simulink model "Linear_Single_Model"  (R2022b)
settings: Solver=FixedStepAuto  StartTime=0.0  StopTime=10.0  FixedStep=0.01  RelTol=1e-3
values from neighbouring files (symbols this model uses):
  V = 30    [linearsinglemodel.m]
settings Model: Creator=FATMANURATA  LastModifiedBy=FATMANURATA

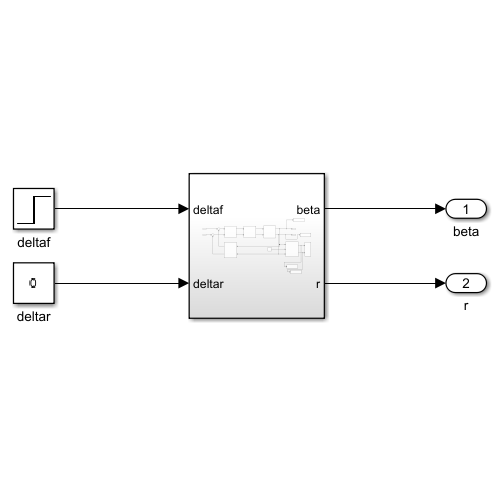
[thumbnail: Simulink's stored preview of the top-level diagram]
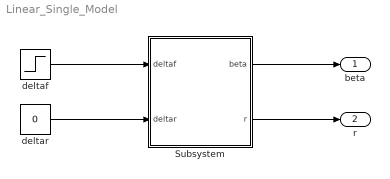
== system Linear_Single_Model ==
  Subsystem : Subsystem
  deltaf : Step  Time=0  SampleTime=0
  deltar : Constant  Value=0
  beta : Outport
  r : Outport  Port=2
  wires:
  deltaf/1 -> Subsystem/1(deltaf)
  deltar/1 -> Subsystem/2(deltar)
  Subsystem/1(beta) -> beta/1
  Subsystem/2(r) -> r/1

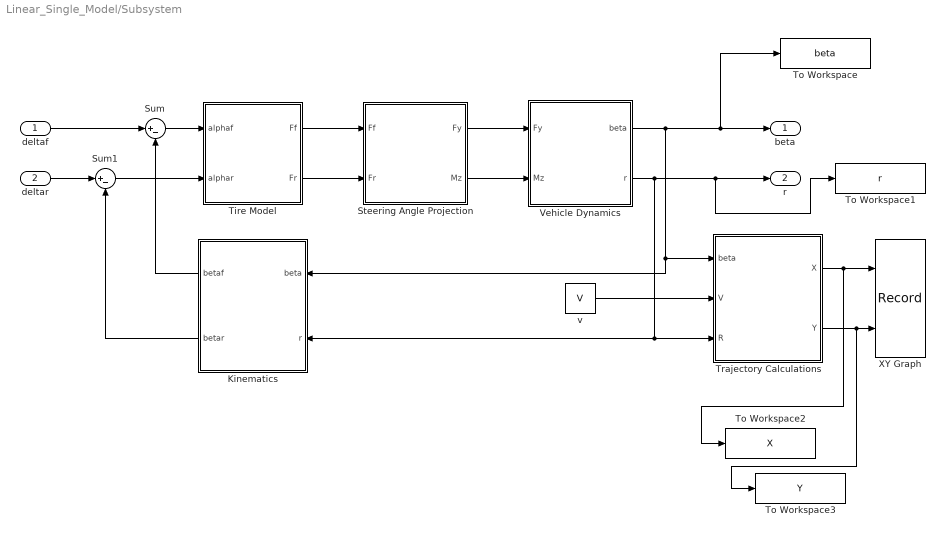
== system Linear_Single_Model/Subsystem ==
  deltaf : Inport
  deltar : Inport  Port=2
  Kinematics : Subsystem
  Steering Angle Projection : Subsystem
  Sum : Sum  Inputs=|+-
  Sum1 : Sum  Inputs=|+-
  Tire Model : Subsystem
  To Workspace : ToWorkspace  VariableName=beta  SampleTime=-1
  To Workspace1 : ToWorkspace  VariableName=r  SampleTime=-1
  To Workspace2 : ToWorkspace  VariableName=X  SampleTime=-1
  To Workspace3 : ToWorkspace  VariableName=Y  SampleTime=-1
  Trajectory Calculations : Subsystem
  Vehicle Dynamics : Subsystem
  XY Graph : Record  FileSettingsInternal="{\"entries\":[{\"content\":{\"excelSettings\":{\"content\":{},\"type\":\"Streamout.ExcelSettings\"}},\"type\":\"Streamout.FileSettingStorage\",\"uuid\":\"eae091c3-533e-4973-b4c9-77a1417e7f04\"}],\"packageUris\":[\"http://schema.mathworks.com/mf0/streamout_blocks/R2020a\"],\"version\":\"1.0\"}"  Layout=[1 1]  SignalsInternal="{\"entries\":[{\"content\":{\"signals\":[{\"content\":{\"blockPath\":[\"Linear_Single_Model/Subsystem/XY Graph\"],\"channel\":[],\"dimensions\":[1],\"domain\":\"Linear_Single_Model/Subsystem/XY Graph\",\"lineColor\":\"#b746ff\",\"plots\":[],\"port\":1,\"sid\":[\"\"],\"signalID\":1937,\"signalName\":\"Trajectory Calculations:1\"},\"type\":\"RecordBlkView.Signal\",\"uuid\":\"180f1f63-cad5-442e-bf7e-af3f779780d9\"},{\"content\":{\"blockPath\":[\"Linear_Single_Model/Subsystem/XY Graph\"],\"channel\":[],\"dimensions\":[1],\"domain\":\"Linear_Single_Model/Subsystem/XY Graph\",\"lineColor\":\"#64d413\",\"plots\":[],\"port\":2,\"sid\":[\"\"],\"signalID\":1941,\"signalName\":\"Trajectory Calculations:2\"},\"type\":\"RecordBlkView.Signal\",\"uuid\":\"a40823eb-ffdd-4da1-8b1e-2047577bc852\"}]},\"type\":\"RecordBlkView.InputSignals\",\"uuid\":\"48f76a04-1f1f-4550-9cf4-1edf313e7d14\"}],\"packageUris\":[\"http://schema.mathworks.com/mf0/streamout_blocks/R2020a\"],\"version\":\"1.0\"}"  VisualizationBindings="{\"xyplotplugin\":{\"info\":[{\"series\":[],\"subplotID\":1}]}}"  CompatibilityTag=XY
  v : Constant  Value=V
  beta : Outport
  r : Outport  Port=2
  wires:
  Kinematics/1(betaf) -> Sum/2
  Trajectory Calculations/2(Y) -> To Workspace3/1, XY Graph/2
  Steering Angle Projection/2(Mz) -> Vehicle Dynamics/2(Mz)
  Vehicle Dynamics/2(r) -> Kinematics/2(r), Trajectory Calculations/3(R), r/1, To Workspace1/1
  Trajectory Calculations/1(X) -> To Workspace2/1, XY Graph/1
  Vehicle Dynamics/1(beta) -> Kinematics/1(beta), Trajectory Calculations/1(beta), beta/1, To Workspace/1
  Sum1/1 -> Tire Model/2(alphar)
  deltar/1 -> Sum1/1
  Tire Model/2(Fr) -> Steering Angle Projection/2(Fr)
  Kinematics/2(betar) -> Sum1/2
  Steering Angle Projection/1(Fy) -> Vehicle Dynamics/1(Fy)
  Sum/1 -> Tire Model/1(alphaf)
  Tire Model/1(Ff) -> Steering Angle Projection/1(Ff)
  v/1 -> Trajectory Calculations/2(V)
  deltaf/1 -> Sum/1

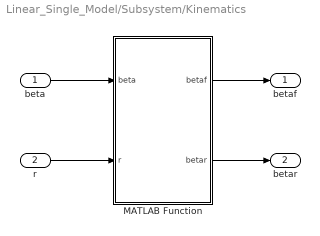
== system Linear_Single_Model/Subsystem/Kinematics ==
  beta : Inport
  r : Inport  Port=2
  MATLAB Function : MATLAB Function  TreatAsAtomicUnit=on
  betaf : Outport
  betar : Outport  Port=2
  wires:
  beta/1 -> MATLAB Function/1(beta)
  r/1 -> MATLAB Function/2(r)
  MATLAB Function/1(betaf) -> betaf/1
  MATLAB Function/2(betar) -> betar/1

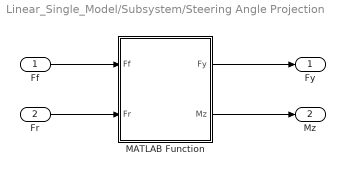
== system Linear_Single_Model/Subsystem/Steering Angle Projection ==
  Ff : Inport
  Fr : Inport  Port=2
  MATLAB Function : MATLAB Function  TreatAsAtomicUnit=on
  Fy : Outport
  Mz : Outport  Port=2
  wires:
  Ff/1 -> MATLAB Function/1(Ff)
  Fr/1 -> MATLAB Function/2(Fr)
  MATLAB Function/1(Fy) -> Fy/1
  MATLAB Function/2(Mz) -> Mz/1

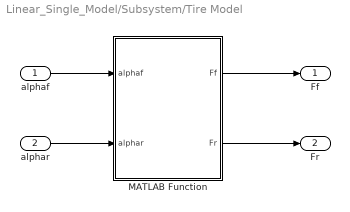
== system Linear_Single_Model/Subsystem/Tire Model ==
  alphaf : Inport
  alphar : Inport  Port=2
  MATLAB Function : MATLAB Function  TreatAsAtomicUnit=on
  Ff : Outport
  Fr : Outport  Port=2
  wires:
  alphaf/1 -> MATLAB Function/1(alphaf)
  alphar/1 -> MATLAB Function/2(alphar)
  MATLAB Function/1(Ff) -> Ff/1
  MATLAB Function/2(Fr) -> Fr/1

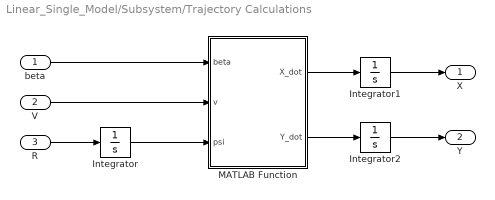
== system Linear_Single_Model/Subsystem/Trajectory Calculations ==
  beta : Inport
  V : Inport  Port=2
  R : Inport  Port=3
  Integrator : Integrator
  Integrator1 : Integrator
  Integrator2 : Integrator
  MATLAB Function : MATLAB Function  TreatAsAtomicUnit=on
  X : Outport
  Y : Outport  Port=2
  wires:
  Integrator/1 -> MATLAB Function/3(psi)
  R/1 -> Integrator/1
  beta/1 -> MATLAB Function/1(beta)
  MATLAB Function/1(X_dot) -> Integrator1/1
  Integrator1/1 -> X/1
  Integrator2/1 -> Y/1
  MATLAB Function/2(Y_dot) -> Integrator2/1
  V/1 -> MATLAB Function/2(v)

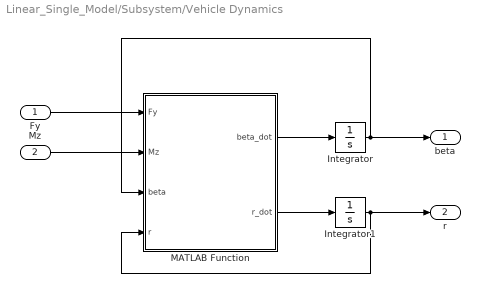
== system Linear_Single_Model/Subsystem/Vehicle Dynamics ==
  Fy : Inport
  Mz : Inport  Port=2
  Integrator : Integrator
  Integrator1 : Integrator
  MATLAB Function : MATLAB Function  TreatAsAtomicUnit=on
  beta : Outport
  r : Outport  Port=2
  wires:
  Fy/1 -> MATLAB Function/1(Fy)
  Mz/1 -> MATLAB Function/2(Mz)
  MATLAB Function/1(beta_dot) -> Integrator/1
  Integrator/1 -> MATLAB Function/3(beta), beta/1
  MATLAB Function/2(r_dot) -> Integrator1/1
  Integrator1/1 -> MATLAB Function/4(r), r/1

== matlab function Linear_Single_Model/Subsystem/Steering Angle Projection/MATLAB Function ==
  data: Ff input; Fy output; Fr input; Mz output
function [Fy, Mz] = fcn(Ff, Fr)
    lf = 1.1; 
    lr = 1.6;

    % Küçük direksiyon açısı kabulü ile sadeleşmiş formüller
    Fy = Ff + Fr;
    Mz = lf * Ff - lr * Fr;
end

== matlab function Linear_Single_Model/Subsystem/Tire Model/MATLAB Function ==
  data: alphaf input; Ff output; alphar input; Fr output
function [Ff, Fr] = fcn(alphaf,alphar)
    cfo = 80000; 

    % Lastik kuvvetleri
    Ff = cfo * alphaf;
    Fr = cfo * alphar;
end

== matlab function Linear_Single_Model/Subsystem/Vehicle Dynamics/MATLAB Function ==
  data: Fy input; beta_dot output; Mz input; beta input; r input; r_dot output
function [beta_dot, r_dot] = fcn(Fy, Mz, beta, r)
    m = 1500;
    J = 2500;
    v = 30; % Hızı buradan sabit olarak alıyoruz (Giriş portu yoksa)

    % r_dot (Yaw acceleration)
    r_dot = Mz / J;

    % beta_dot (Side-slip rate)
    beta_dot = (Fy / (m * v)) - r;
end

== matlab function Linear_Single_Model/Subsystem/Trajectory Calculations/MATLAB Function ==
  data: beta input; X_dot output; v input; psi input; Y_dot output
function [X_dot, Y_dot] = fcn(beta, v, psi)
    X_dot = v * cos(beta + psi);
    Y_dot = v * sin(beta + psi);
end

== matlab function Linear_Single_Model/Subsystem/Kinematics/MATLAB Function ==
  data: beta input; betaf output; r input; betar output
function [betaf, betar] = fcn(beta, r)
    lf = 1.1; 
    lr = 1.6;
    v = 30; % Hızı burada sabit tanımlıyoruz (Kablo çekmediğin için)

    % Linear formüller (Küçük açı kabulü)
    betaf = beta + (r * lf) / v;
    betar = beta - (r * lr) / v;
end
